simulink model "closeLoopSimulation"  (R2024a)
settings: Solver=VariableStepAuto  StartTime=0.0  StopTime=10000  RelTol=1e-3
undefined symbols (not defined in the file or in its folder): Error_quaternio, feedback, init, motor, sat, setPoint
libraries: aerolibconvert2 x2, sharedtransform x2
settings Model: Creator=b_ant  LastModifiedBy=b_ant
settings DataIOCC: SaveFormat=Array

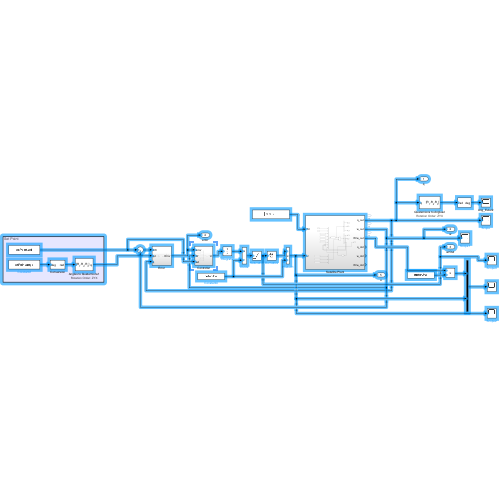
[thumbnail: Simulink's stored preview of the top-level diagram]
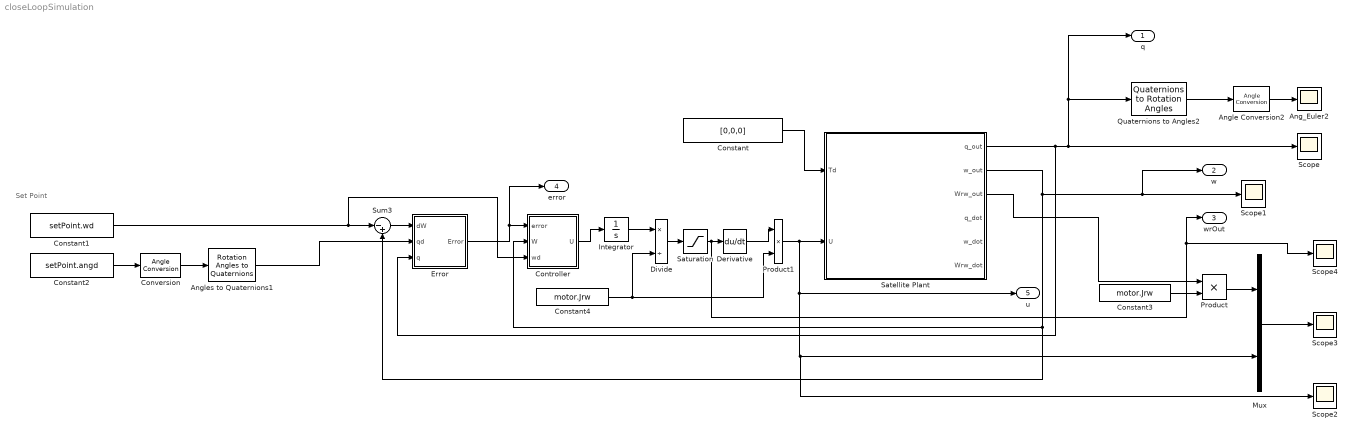
== system closeLoopSimulation ==
  note: Set Point
  Ang_Euler2 : Scope
  Angle Conversion2 : aerolibconvert2/Angle Conversion  IU=rad  OU=deg
  Angles to Quaternions1 : sharedtransform/Rotation Angles to Quaternions  rotationOrder=ZYX  aMode=aMode
  Constant : Constant  Value=[0,0,0]
  Constant1 : Constant  Value=setPoint.wd
  Constant2 : Constant  Value=setPoint.angd
  Constant3 : Constant  Value=motor.Jrw
  Constant4 : Constant  Value=motor.Jrw
  Controller : Subsystem
  Conversion : aerolibconvert2/Angle Conversion  IU=deg  OU=rad
  Derivative : Derivative
  Divide : Product  Inputs=*/
  Error : Subsystem
  Integrator : Integrator
  Mux : Mux  Inputs=2
  Product : Product
  Product1 : Product
  Quaternions to Angles2 : sharedtransform/Quaternions to Rotation Angles  rotationOrder=ZYX  aMode=aMode
  Satellite Plant : Subsystem
  Saturation : Saturate  UpperLimit=457.6253298729  LowerLimit=-457.6253298729
  Scope{,1..4} (5 alike) : Scope
  Sum3 : Sum  Inputs=|-+
  q : Outport
  w : Outport  Port=2
  wrOut : Outport  Port=3
  error : Outport  Port=4
  u : Outport  Port=5
  wires:
  Constant/1 -> Satellite Plant/1(Td)
  Constant1/1 -> Sum3/1, Controller/3(wd)
  Conversion/1 -> Angles to Quaternions1/1
  Constant2/1 -> Conversion/1
  Satellite Plant/1(q_out) -> q/1, Quaternions to Angles2/1, Scope/1, Error/3(q)
  Quaternions to Angles2/1 -> Angle Conversion2/1
  Angle Conversion2/1 -> Ang_Euler2/1
  Sum3/1 -> Error/1(dW)
  Angles to Quaternions1/1 -> Error/2(qd)
  Error/1(Error) -> Controller/1(error), error/1
  Satellite Plant/2(w_out) -> Sum3/2, Controller/2(W), w/1, Scope1/1
  Satellite Plant/3(Wrw_out) -> Product/1
  Constant3/1 -> Product/2
  Product/1 -> Mux/1
  Mux/1 -> Scope3/1
  Controller/1(U) -> Integrator/1
  Integrator/1 -> Divide/1
  Constant4/1 -> Product1/2, Divide/2
  Divide/1 -> Saturation/1
  Saturation/1 -> Scope4/1, wrOut/1, Derivative/1
  Derivative/1 -> Product1/1
  Product1/1 -> Scope2/1, Mux/2, u/1, Satellite Plant/2(U)

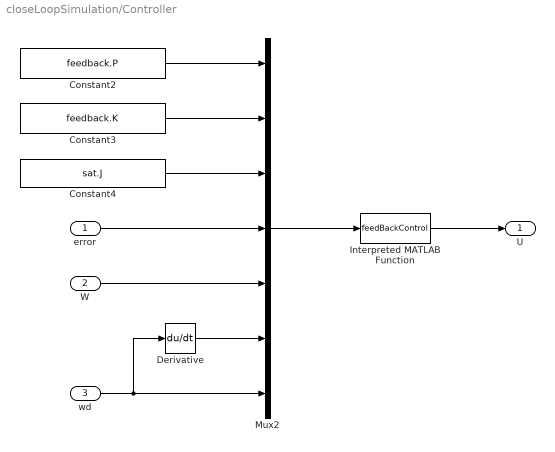
== system closeLoopSimulation/Controller ==
  error : Inport
  W : Inport  Port=2
  wd : Inport  Port=3
  Constant2 : Constant  Value=feedback.P
  Constant3 : Constant  Value=feedback.K
  Constant4 : Constant  Value=sat.J
  Derivative : Derivative
  Interpreted MATLAB Function : MATLABFcn  MATLABFcn=feedBackControl  OutputDimensions=3
  Mux2 : Mux  Inputs=7
  U : Outport
  wires:
  Interpreted MATLAB Function/1 -> U/1
  Constant2/1 -> Mux2/1
  Mux2/1 -> Interpreted MATLAB Function/1
  W/1 -> Mux2/5
  Constant3/1 -> Mux2/2
  error/1 -> Mux2/4
  Constant4/1 -> Mux2/3
  Derivative/1 -> Mux2/6
  wd/1 -> Derivative/1, Mux2/7

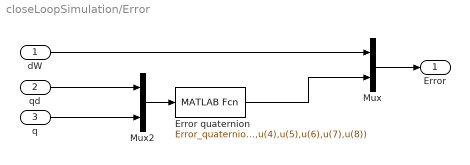
== system closeLoopSimulation/Error ==
  dW : Inport
  qd : Inport  Port=2
  q : Inport  Port=3
  Error quaternion : MATLABFcn  MATLABFcn=Error_quaternio(u(1),u(2),u(3),u(4),u(5),u(6),u(7),u(8))
  Mux : Mux  Inputs=2
  Mux2 : Mux  Inputs=2
  Error : Outport
  wires:
  Error quaternion/1 -> Mux/2
  Mux2/1 -> Error quaternion/1
  q/1 -> Mux2/2
  dW/1 -> Mux/1
  qd/1 -> Mux2/1
  Mux/1 -> Error/1

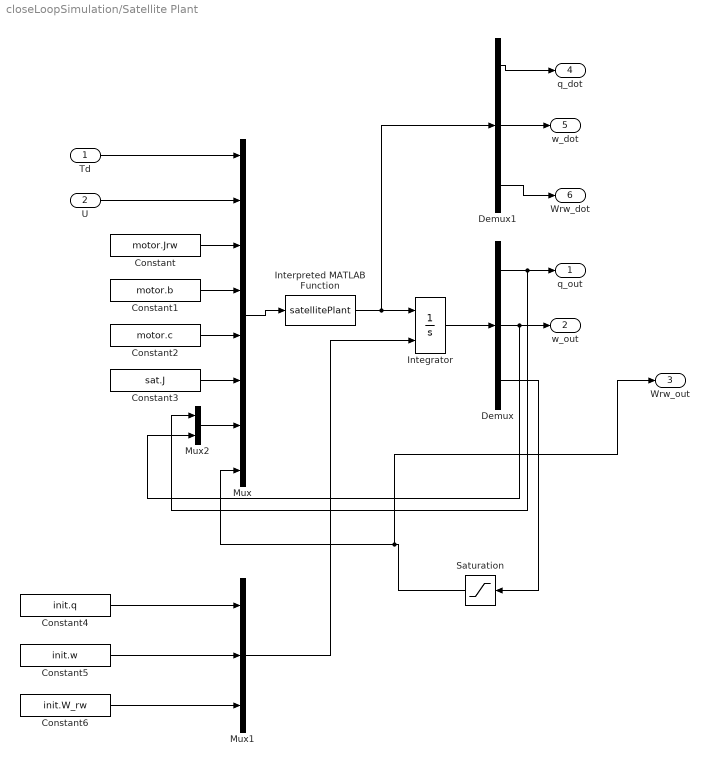
== system closeLoopSimulation/Satellite Plant ==
  Td : Inport
  U : Inport  Port=2
  Constant : Constant  Value=motor.Jrw
  Constant1 : Constant  Value=motor.b
  Constant2 : Constant  Value=motor.c
  Constant3 : Constant  Value=sat.J
  Constant4 : Constant  Value=init.q
  Constant5 : Constant  Value=init.w
  Constant6 : Constant  Value=init.W_rw
  Demux : Demux  Outputs=3
  Demux1 : Demux  Outputs=3
  Integrator : Integrator  InitialConditionSource=external
  Interpreted MATLAB Function : MATLABFcn  MATLABFcn=satellitePlant
  Mux : Mux  Inputs=8
  Mux1 : Mux  Inputs=3
  Mux2 : Mux  Inputs=2
  Saturation : Saturate  UpperLimit=457.6253298729  LowerLimit=-457.6253298729
  q_out : Outport
  w_out : Outport  Port=2
  Wrw_out : Outport  Port=3
  q_dot : Outport  Port=4
  w_dot : Outport  Port=5
  Wrw_dot : Outport  Port=6
  wires:
  Td/1 -> Mux/1
  Mux/1 -> Interpreted MATLAB Function/1
  U/1 -> Mux/2
  Interpreted MATLAB Function/1 -> Demux1/1, Integrator/1
  Constant/1 -> Mux/3
  Constant5/1 -> Mux1/2
  Constant6/1 -> Mux1/3
  Constant4/1 -> Mux1/1
  Mux1/1 -> Integrator/2
  Constant1/1 -> Mux/4
  Constant2/1 -> Mux/5
  Constant3/1 -> Mux/6
  Integrator/1 -> Demux/1
  Demux/1 -> Mux2/1, q_out/1
  Demux/2 -> Mux2/2, w_out/1
  Demux/3 -> Saturation/1
  Demux1/3 -> Wrw_dot/1
  Demux1/1 -> q_dot/1
  Demux1/2 -> w_dot/1
  Mux2/1 -> Mux/7
  Saturation/1 -> Wrw_out/1, Mux/8
